simulink model "Scenario_13_CoDeSys"  (R2012b)
settings: Solver=ode3  StartTime=0.0  StopTime=inf  FixedStep=Sample_Time_Model  RelTol=1e-3
PreLoadFcn:
  | Variablen_Scenario13
InitFcn:
  | BT = randperm(9);
values from neighbouring files (symbols this model uses):
  Band_Geschwindigkeit = 1.47    [Variablen_Scenario13.m]
  Band_Sensor_Hell_2_Z = -6.5    [Variablen_Scenario13.m]
  Band_Sensor_Hell_3_Z = -10.36    [Variablen_Scenario13.m]
  Band_Sensor_Hell_4_Z = -14.64    [Variablen_Scenario13.m]
  Band_Sensor_Tolerance_Z = 0.2    [Variablen_Scenario13.m]
  Bauteil_Fallgeschwindigkeit = 0.4    [Variablen_Scenario13.m]
  Bauteil_Farbe_Metall = [0.8 0.8 0.8]    [Variablen_Scenario13.m]
  Bauteil_Farbe_Schwarz = [0.2 0.2 0.2]    [Variablen_Scenario13.m]
  Bauteil_Farbe_Weiss = [1 1 0.2]    [Variablen_Scenario13.m]
  Kran_Dauer_90_Grad = 5    [Variablen_Scenario13.m]
  Kran_Drehwinkel_90_Grad = 8050    [Variablen_Scenario13.m]
  Kran_Sensor_Position_Delta = 0.07    [Variablen_Scenario13.m]
  Sample_Time_Model = 0.05    [Variablen_Scenario13.m]
  Sample_Time_Simulation = 0.1    [Variablen_Scenario13.m]
  Sensor_Band_Metall_1 = -6.5    [Variablen_Scenario13.m]
  Sensor_Band_Metall_2 = -10.36    [Variablen_Scenario13.m]
libraries: simulink x557, vrlib x13, opclib x7, rtwinlib x1
(part 5 of 10)

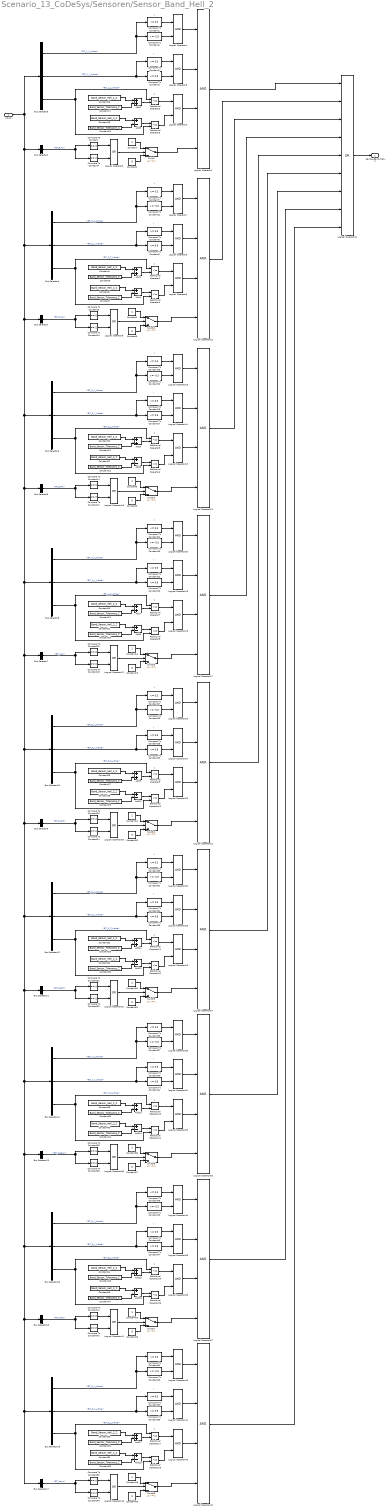
== system Scenario_13_CoDeSys/Sensoren/Sensor_Band_Hell_2 ==
  note: Y
  note: X
  note: Z
  note: Y
  note: X
  note: Z
  note: Y
  note: X
  note: Z
  note: Y
  note: X
  note: Z
  note: Y
  note: X
  note: Z
  note: Y
  note: X
  note: Z
  note: Y
  note: Z
  note: Y
  note: Z
  note: Y
  note: Z
  Inputs : Inport
  Add{1..2,5,7,9,11,13,15,17} (9 alike) : Sum
  Add{3..4,6,8,10,12,14,16,18} (9 alike) : Sum  Inputs=+-
  Bus Selector1 : BusSelector  OutputSignals=Eingaenge.Bauteile.BT_Zwei
  Bus Selector10 : BusSelector  OutputSignals=Bauteil.Stempelanlage_BT.Bauteil_5.BT_5_X_Achse,Bauteil.Stempelanlage_BT.Bauteil_5.BT_5_Y_Achse,Bauteil.Stempelanlage_BT.Bauteil_5.BT_5_Z_Achse
  Bus Selector11 : BusSelector  OutputSignals=Eingaenge.Bauteile.BT_Sechs
  Bus Selector12 : BusSelector  OutputSignals=Bauteil.Stempelanlage_BT.Bauteil_6.BT_6_X_Achse,Bauteil.Stempelanlage_BT.Bauteil_6.BT_6_Y_Achse,Bauteil.Stempelanlage_BT.Bauteil_6.BT_6_Z_Achse
  Bus Selector13 : BusSelector  OutputSignals=Eingaenge.Bauteile.BT_Sieben
  Bus Selector14 : BusSelector  OutputSignals=Bauteil.Stempelanlage_BT.Bauteil_7.BT_7_X_Achse,Bauteil.Stempelanlage_BT.Bauteil_7.BT_7_Y_Achse,Bauteil.Stempelanlage_BT.Bauteil_7.BT_7_Z_Achse
  Bus Selector15 : BusSelector  OutputSignals=Eingaenge.Bauteile.BT_Acht
  Bus Selector16 : BusSelector  OutputSignals=Bauteil.Stempelanlage_BT.Bauteil_8.BT_8_X_Achse,Bauteil.Stempelanlage_BT.Bauteil_8.BT_8_Y_Achse,Bauteil.Stempelanlage_BT.Bauteil_8.BT_8_Z_Achse
  Bus Selector17 : BusSelector  OutputSignals=Eingaenge.Bauteile.BT_Neun
  Bus Selector18 : BusSelector  OutputSignals=Bauteil.Stempelanlage_BT.Bauteil_9.BT_9_X_Achse,Bauteil.Stempelanlage_BT.Bauteil_9.BT_9_Y_Achse,Bauteil.Stempelanlage_BT.Bauteil_9.BT_9_Z_Achse
  Bus Selector2 : BusSelector  OutputSignals=Eingaenge.Bauteile.BT_Eins
  Bus Selector3 : BusSelector  OutputSignals=Bauteil.Stempelanlage_BT.Bauteil_1.BT_1_X_Achse,Bauteil.Stempelanlage_BT.Bauteil_1.BT_1_Y_Achse,Bauteil.Stempelanlage_BT.Bauteil_1.BT_1_Z_Achse
  Bus Selector4 : BusSelector  OutputSignals=Bauteil.Stempelanlage_BT.Bauteil_2.BT_2_X_Achse,Bauteil.Stempelanlage_BT.Bauteil_2.BT_2_Y_Achse,Bauteil.Stempelanlage_BT.Bauteil_2.BT_2_Z_Achse
  Bus Selector5 : BusSelector  OutputSignals=Eingaenge.Bauteile.BT_Drei
  Bus Selector6 : BusSelector  OutputSignals=Bauteil.Stempelanlage_BT.Bauteil_3.BT_3_X_Achse,Bauteil.Stempelanlage_BT.Bauteil_3.BT_3_Y_Achse,Bauteil.Stempelanlage_BT.Bauteil_3.BT_3_Z_Achse
  Bus Selector7 : BusSelector  OutputSignals=Eingaenge.Bauteile.BT_Vier
  Bus Selector8 : BusSelector  OutputSignals=Bauteil.Stempelanlage_BT.Bauteil_4.BT_4_X_Achse,Bauteil.Stempelanlage_BT.Bauteil_4.BT_4_Y_Achse,Bauteil.Stempelanlage_BT.Bauteil_4.BT_4_Z_Achse
  Bus Selector9 : BusSelector  OutputSignals=Eingaenge.Bauteile.BT_Fuenf
  Compare To Constant{,5,14,20,26,32,38,44,50} (9 alike) : simulink/Logic and Bit Operations/Compare To Constant  relop===  const=0  OutDataTypeStr=boolean
  Compare To Constant{1,7,15,21,27,33,39,45,51} (9 alike) : simulink/Logic and Bit Operations/Compare To Constant  relop=<=  const=0.3  OutDataTypeStr=boolean
  Compare To Constant{4,10,12,18,24,30,36,42,48} (9 alike) : simulink/Logic and Bit Operations/Compare To Constant  relop===  const=2  OutDataTypeStr=boolean
  Compare To Constant{6,11,13,19,25,31,37,43,49} (9 alike) : simulink/Logic and Bit Operations/Compare To Constant  relop=>=  const=-0.3  OutDataTypeStr=boolean
  Compare To Constant{2,8,16,22,28,34,40,46,52} (9 alike) : simulink/Logic and Bit Operations/Compare To Constant  relop=>=  const=0.5  OutDataTypeStr=boolean
  Compare To Constant{3,9,17,23,29,35,41,47,53} (9 alike) : simulink/Logic and Bit Operations/Compare To Constant  relop=<=  const=0.9  OutDataTypeStr=boolean
  Constant{,2,8,14,24,30,36,42,48} (9 alike) : Constant
  Constant{1,3,9,15,25,31,37,43,49} (9 alike) : Constant  Value=0
  Constant{4,6,10,12,16,18,20,22,26,28,32,34,38,40,44,46,50,52} (18 alike) : Constant  Value=Band_Sensor_Hell_2_Z
  Constant{5,7,11,13,17,19,21,23,27,29,33,35,39,41,45,47,51,53} (18 alike) : Constant  Value=Band_Sensor_Tolerance_Z
  Logical Operator{1,10,12,17,22,27,32,37,42} (9 alike) : Logic  Inputs=4  AllPortsSameDT=off  OutDataTypeStr=boolean
  Logical Operator11 : Logic  Operator=OR  Inputs=9  AllPortsSameDT=off  OutDataTypeStr=boolean
  Logical Operator{2..7,13..15,18..20,23..25,28..30,33..35,38..40,43..45} (27 alike) : Logic  AllPortsSameDT=off  OutDataTypeStr=boolean
  Logical Operator{8..9,16,21,26,31,36,41,46} (9 alike) : Logic  Operator=OR  AllPortsSameDT=off  OutDataTypeStr=boolean
  Relational Operator{1..18} (18 alike) : RelationalOperator  Operator=<=  OutDataTypeStr=boolean
  Switch{,1..8} (9 alike) : Switch  Threshold=1
  Sensor_Band_Hell_2 : Outport
  wires:
  Bus Selector3/2 -> Compare To Constant2/1, Compare To Constant3/1  "<BT_1_Y_Achse>"
  Compare To Constant2/1 -> Logical Operator3/1
  Compare To Constant3/1 -> Logical Operator3/2
  Logical Operator3/1 -> Logical Operator1/2
  Logical Operator2/1 -> Logical Operator1/3
  Bus Selector3/1 -> Compare To Constant1/1, Compare To Constant6/1  "<BT_1_X_Achse>"
  Compare To Constant1/1 -> Logical Operator4/1
  Compare To Constant6/1 -> Logical Operator4/2
  Logical Operator4/1 -> Logical Operator1/1
  Bus Selector2/1 -> Compare To Constant/1, Compare To Constant4/1  "<BT_Eins>"
  Constant/1 -> Switch/1
  Constant1/1 -> Switch/3
  Relational Operator2/1 -> Logical Operator2/1
  Constant16/1 -> Add2/1
  Constant17/1 -> Add2/2
  Constant18/1 -> Add3/1
  Constant19/1 -> Add3/2
  Add2/1 -> Relational Operator2/2
  Add3/1 -> Relational Operator3/1
  Bus Selector3/3 -> Relational Operator2/1, Relational Operator3/2  "<BT_1_Z_Achse>"
  Relational Operator3/1 -> Logical Operator2/2
  Compare To Constant/1 -> Logical Operator9/1
  Compare To Constant4/1 -> Logical Operator9/2
  Logical Operator9/1 -> Switch/2
  Switch/1 -> Logical Operator1/4
  Compare To Constant8/1 -> Logical Operator6/1
  Compare To Constant9/1 -> Logical Operator6/2
  Logical Operator6/1 -> Logical Operator10/2
  Logical Operator5/1 -> Logical Operator10/3
  Bus Selector4/1 -> Compare To Constant7/1, Compare To Constant11/1  "<BT_2_X_Achse>"
  Compare To Constant7/1 -> Logical Operator7/1
  Compare To Constant11/1 -> Logical Operator7/2
  Logical Operator7/1 -> Logical Operator10/1
  Bus Selector1/1 -> Compare To Constant5/1, Compare To Constant10/1  "<BT_Zwei>"
  Constant2/1 -> Switch1/1
  Constant3/1 -> Switch1/3
  Relational Operator1/1 -> Logical Operator5/1
  Constant4/1 -> Add1/1
  Constant5/1 -> Add1/2
  Constant6/1 -> Add4/1
  Constant7/1 -> Add4/2
  Add1/1 -> Relational Operator1/2
  Add4/1 -> Relational Operator4/1
  Bus Selector4/3 -> Relational Operator1/1, Relational Operator4/2  "<BT_2_Z_Achse>"
  Relational Operator4/1 -> Logical Operator5/2
  Compare To Constant5/1 -> Logical Operator8/1
  Compare To Constant10/1 -> Logical Operator8/2
  Logical Operator8/1 -> Switch1/2
  Switch1/1 -> Logical Operator10/4
  Bus Selector4/2 -> Compare To Constant8/1, Compare To Constant9/1  "<BT_2_Y_Achse>"
  Logical Operator11/1 -> Sensor_Band_Hell_2/1
  Logical Operator1/1 -> Logical Operator11/1
  Logical Operator10/1 -> Logical Operator11/2
  Compare To Constant16/1 -> Logical Operator14/1
  Compare To Constant17/1 -> Logical Operator14/2
  Logical Operator14/1 -> Logical Operator12/2
  Logical Operator13/1 -> Logical Operator12/3
  Bus Selector6/1 -> Compare To Constant15/1, Compare To Constant13/1  "<BT_3_X_Achse>"
  Compare To Constant15/1 -> Logical Operator15/1
  Compare To Constant13/1 -> Logical Operator15/2
  Logical Operator15/1 -> Logical Operator12/1
  Bus Selector5/1 -> Compare To Constant14/1, Compare To Constant12/1  "<BT_Drei>"
  Constant8/1 -> Switch2/1
  Constant9/1 -> Switch2/3
  Relational Operator5/1 -> Logical Operator13/1
  Constant10/1 -> Add5/1
  Constant11/1 -> Add5/2
  Constant12/1 -> Add6/1
  Constant13/1 -> Add6/2
  Add5/1 -> Relational Operator5/2
  Add6/1 -> Relational Operator6/1
  Bus Selector6/3 -> Relational Operator5/1, Relational Operator6/2  "<BT_3_Z_Achse>"
  Relational Operator6/1 -> Logical Operator13/2
  Compare To Constant14/1 -> Logical Operator16/1
  Compare To Constant12/1 -> Logical Operator16/2
  Logical Operator16/1 -> Switch2/2
  Switch2/1 -> Logical Operator12/4
  Bus Selector6/2 -> Compare To Constant16/1, Compare To Constant17/1  "<BT_3_Y_Achse>"
  Compare To Constant22/1 -> Logical Operator19/1
  Compare To Constant23/1 -> Logical Operator19/2
  Logical Operator19/1 -> Logical Operator17/2
  Logical Operator18/1 -> Logical Operator17/3
  Bus Selector8/1 -> Compare To Constant21/1, Compare To Constant19/1  "<BT_4_X_Achse>"
  Compare To Constant21/1 -> Logical Operator20/1
  Compare To Constant19/1 -> Logical Operator20/2
  Logical Operator20/1 -> Logical Operator17/1
  Bus Selector7/1 -> Compare To Constant20/1, Compare To Constant18/1  "<BT_Vier>"
  Constant14/1 -> Switch3/1
  Constant15/1 -> Switch3/3
  Relational Operator7/1 -> Logical Operator18/1
  Constant20/1 -> Add7/1
  Constant21/1 -> Add7/2
  Constant22/1 -> Add8/1
  Constant23/1 -> Add8/2
  Add7/1 -> Relational Operator7/2
  Add8/1 -> Relational Operator8/1
  Bus Selector8/3 -> Relational Operator7/1, Relational Operator8/2  "<BT_4_Z_Achse>"
  Relational Operator8/1 -> Logical Operator18/2
  Compare To Constant20/1 -> Logical Operator21/1
  Compare To Constant18/1 -> Logical Operator21/2
  Logical Operator21/1 -> Switch3/2
  Switch3/1 -> Logical Operator17/4
  Bus Selector8/2 -> Compare To Constant22/1, Compare To Constant23/1  "<BT_4_Y_Achse>"
  Compare To Constant28/1 -> Logical Operator24/1
  Compare To Constant29/1 -> Logical Operator24/2
  Logical Operator24/1 -> Logical Operator22/2
  Logical Operator23/1 -> Logical Operator22/3
  Bus Selector10/1 -> Compare To Constant27/1, Compare To Constant25/1  "<BT_5_X_Achse>"
  Compare To Constant27/1 -> Logical Operator25/1
  Compare To Constant25/1 -> Logical Operator25/2
  Logical Operator25/1 -> Logical Operator22/1
  Bus Selector9/1 -> Compare To Constant26/1, Compare To Constant24/1  "<BT_Fuenf>"
  Constant24/1 -> Switch4/1
  Constant25/1 -> Switch4/3
  Relational Operator9/1 -> Logical Operator23/1
  Constant26/1 -> Add9/1
  Constant27/1 -> Add9/2
  Constant28/1 -> Add10/1
  Constant29/1 -> Add10/2
  Add9/1 -> Relational Operator9/2
  Add10/1 -> Relational Operator10/1
  Bus Selector10/3 -> Relational Operator9/1, Relational Operator10/2  "<BT_5_Z_Achse>"
  Relational Operator10/1 -> Logical Operator23/2
  Compare To Constant26/1 -> Logical Operator26/1
  Compare To Constant24/1 -> Logical Operator26/2
  Logical Operator26/1 -> Switch4/2
  Switch4/1 -> Logical Operator22/4
  Bus Selector10/2 -> Compare To Constant28/1, Compare To Constant29/1  "<BT_5_Y_Achse>"
  Compare To Constant34/1 -> Logical Operator29/1
  Compare To Constant35/1 -> Logical Operator29/2
  Logical Operator29/1 -> Logical Operator27/2
  Logical Operator28/1 -> Logical Operator27/3
  Bus Selector12/1 -> Compare To Constant33/1, Compare To Constant31/1  "<BT_6_X_Achse>"
  Compare To Constant33/1 -> Logical Operator30/1
  Compare To Constant31/1 -> Logical Operator30/2
  Logical Operator30/1 -> Logical Operator27/1
  Bus Selector11/1 -> Compare To Constant32/1, Compare To Constant30/1  "<BT_Sechs>"
  Constant30/1 -> Switch5/1
  Constant31/1 -> Switch5/3
  Relational Operator11/1 -> Logical Operator28/1
  Constant32/1 -> Add11/1
  Constant33/1 -> Add11/2
  Constant34/1 -> Add12/1
  Constant35/1 -> Add12/2
  Add11/1 -> Relational Operator11/2
  Add12/1 -> Relational Operator12/1
  Bus Selector12/3 -> Relational Operator11/1, Relational Operator12/2  "<BT_6_Z_Achse>"
  Relational Operator12/1 -> Logical Operator28/2
  Compare To Constant32/1 -> Logical Operator31/1
  Compare To Constant30/1 -> Logical Operator31/2
  Logical Operator31/1 -> Switch5/2
  Switch5/1 -> Logical Operator27/4
  Bus Selector12/2 -> Compare To Constant34/1, Compare To Constant35/1  "<BT_6_Y_Achse>"
  Logical Operator12/1 -> Logical Operator11/3
  Logical Operator17/1 -> Logical Operator11/4
  Logical Operator22/1 -> Logical Operator11/5
  Logical Operator27/1 -> Logical Operator11/6
  Inputs/1 -> Bus Selector6/1, Bus Selector5/1, Bus Selector8/1, Bus Selector7/1, Bus Selector10/1, Bus Selector9/1, Bus Selector12/1, Bus Selector14/1, Bus Selector13/1, Bus Selector16/1, Bus Selector15/1, Bus Selector18/1, Bus Selector17/1, Bus Selector11/1, Bus Selector1/1, Bus Selector4/1, Bus Selector2/1, Bus Selector3/1
  Compare To Constant40/1 -> Logical Operator34/1
  Compare To Constant41/1 -> Logical Operator34/2
  Logical Operator34/1 -> Logical Operator32/2
  Logical Operator33/1 -> Logical Operator32/3
  Bus Selector14/1 -> Compare To Constant39/1, Compare To Constant37/1  "<BT_7_X_Achse>"
  Compare To Constant39/1 -> Logical Operator35/1
  Compare To Constant37/1 -> Logical Operator35/2
  Logical Operator35/1 -> Logical Operator32/1
  Bus Selector13/1 -> Compare To Constant38/1, Compare To Constant36/1  "<BT_Sieben>"
  Constant36/1 -> Switch6/1
  Constant37/1 -> Switch6/3
  Relational Operator13/1 -> Logical Operator33/1
  Constant38/1 -> Add13/1
  Constant39/1 -> Add13/2
  Constant40/1 -> Add14/1
  Constant41/1 -> Add14/2
  Add13/1 -> Relational Operator13/2
  Add14/1 -> Relational Operator14/1
  Bus Selector14/3 -> Relational Operator13/1, Relational Operator14/2  "<BT_7_Z_Achse>"
  Relational Operator14/1 -> Logical Operator33/2
  Compare To Constant38/1 -> Logical Operator36/1
  Compare To Constant36/1 -> Logical Operator36/2
  Logical Operator36/1 -> Switch6/2
  Switch6/1 -> Logical Operator32/4
  Bus Selector14/2 -> Compare To Constant40/1, Compare To Constant41/1  "<BT_7_Y_Achse>"
  Compare To Constant46/1 -> Logical Operator39/1
  Compare To Constant47/1 -> Logical Operator39/2
  Logical Operator39/1 -> Logical Operator37/2
  Logical Operator38/1 -> Logical Operator37/3
  Bus Selector16/1 -> Compare To Constant45/1, Compare To Constant43/1  "<BT_8_X_Achse>"
  Compare To Constant45/1 -> Logical Operator40/1
  Compare To Constant43/1 -> Logical Operator40/2
  Logical Operator40/1 -> Logical Operator37/1
  Bus Selector15/1 -> Compare To Constant44/1, Compare To Constant42/1  "<BT_Acht>"
  Constant42/1 -> Switch7/1
  Constant43/1 -> Switch7/3
  Relational Operator15/1 -> Logical Operator38/1
  Constant44/1 -> Add15/1
  Constant45/1 -> Add15/2
  Constant46/1 -> Add16/1
  Constant47/1 -> Add16/2
  Add15/1 -> Relational Operator15/2
  Add16/1 -> Relational Operator16/1
  Bus Selector16/3 -> Relational Operator15/1, Relational Operator16/2  "<BT_8_Z_Achse>"
  Relational Operator16/1 -> Logical Operator38/2
  Compare To Constant44/1 -> Logical Operator41/1
  Compare To Constant42/1 -> Logical Operator41/2
  Logical Operator41/1 -> Switch7/2
  Switch7/1 -> Logical Operator37/4
  Bus Selector16/2 -> Compare To Constant46/1, Compare To Constant47/1  "<BT_8_Y_Achse>"
  Compare To Constant52/1 -> Logical Operator44/1
  Compare To Constant53/1 -> Logical Operator44/2
  Logical Operator44/1 -> Logical Operator42/2
  Logical Operator43/1 -> Logical Operator42/3
  Bus Selector18/1 -> Compare To Constant51/1, Compare To Constant49/1  "<BT_9_X_Achse>"
  Compare To Constant51/1 -> Logical Operator45/1
  Compare To Constant49/1 -> Logical Operator45/2
  Logical Operator45/1 -> Logical Operator42/1
  Bus Selector17/1 -> Compare To Constant48/1, Compare To Constant50/1  "<BT_Neun>"
  Constant48/1 -> Switch8/1
  Constant49/1 -> Switch8/3
  Relational Operator17/1 -> Logical Operator43/1
  Constant50/1 -> Add17/1
  Constant51/1 -> Add17/2
  Constant52/1 -> Add18/1
  Constant53/1 -> Add18/2
  Add17/1 -> Relational Operator17/2
  Add18/1 -> Relational Operator18/1
  Bus Selector18/3 -> Relational Operator17/1, Relational Operator18/2  "<BT_9_Z_Achse>"
  Relational Operator18/1 -> Logical Operator43/2
  Compare To Constant50/1 -> Logical Operator46/1
  Compare To Constant48/1 -> Logical Operator46/2
  Logical Operator46/1 -> Switch8/2
  Switch8/1 -> Logical Operator42/4
  Bus Selector18/2 -> Compare To Constant52/1, Compare To Constant53/1  "<BT_9_Y_Achse>"
  Logical Operator32/1 -> Logical Operator11/7
  Logical Operator37/1 -> Logical Operator11/8
  Logical Operator42/1 -> Logical Operator11/9

== stateflow chart Scenario_13_CoDeSys/Signal Expander/Band_Zyl_1 ==
  state Schrittgroesse [function]
    (default) -> (junction 106) : {Schrittgroesse = (3* Sample_Time)/0.11}
  state Berechne_Naechste_Position_Einfahren [function]
    (default) -> (junction 134) : {Naechste_Position = Zyl_1_X_Achse - Schrittgroesse;}
    (junction 134) -> (junction 135) [order 1] : [Naechste_Position <= -1]
    (junction 134) -> (junction 136) [order 2] : {Zyl_1_X_Achse = Naechste_Position;}
    (junction 135) -> (junction 137) : {Zyl_1_X_Achse = -1;}
    (junction 137) -> (junction 136)
  state Zyl_1_Bereit
    entry: Zyl_1_X_Achse = -1;
    Band_Zyl_1_Eingefahren = 1;
    exit: Band_Zyl_1_Eingefahren = 0;
  state Berechne_Naechste_Position_Ausfahren [function]
    (default) -> (junction 124) : {Naechste_Position = Zyl_1_X_Achse + Schrittgroesse;}
    (junction 124) -> (junction 125) [order 1] : [Naechste_Position >= 2]
    (junction 124) -> (junction 126) [order 2] : {Zyl_1_X_Achse = Naechste_Position;}
    (junction 125) -> (junction 127) : {Zyl_1_X_Achse = 2;}
    (junction 127) -> (junction 126)
  state r = Stop_Einfahren [function]
    (default) -> (junction 198) : {r=0}
    (junction 198) -> (junction 199) [order 1] : [!Zyl_1_Einfahren || (Zyl_1_Ausfahren && Zyl_1_Einfahren)]
    (junction 199) -> (junction 201) : {r=1}
    (junction 198) -> (junction 200) [order 2]
    (junction 201) -> (junction 200)
  state Stop
  state Zyl_1_Ausfahren
    during: Berechne_Naechste_Position_Ausfahren();
  state r = Stop_Ausfahren [function]
    (default) -> (junction 209) : {r=0}
    (junction 209) -> (junction 210) [order 1] : [!Zyl_1_Ausfahren || (Zyl_1_Ausfahren && Zyl_1_Einfahren)]
    (junction 210) -> (junction 212) : {r=1}
    (junction 209) -> (junction 211) [order 2]
    (junction 212) -> (junction 211)
  state r = Continue_Einfahren [function]
    (default) -> (junction 187) : {r=0}
    (junction 187) -> (junction 188) [order 1] : [Zyl_1_Einfahren && !Zyl_1_Ausfahren]
    (junction 188) -> (junction 190) : {r=1}
    (junction 187) -> (junction 189) [order 2]
    (junction 190) -> (junction 189)
  state Zyl_1_Ausgefahren
    entry: Band_Zyl_1_Ausgefahren = 1;
    Zyl_1_X_Achse = 2;
    exit: Band_Zyl_1_Ausgefahren = 0;
  state r = Continue_Ausfahren [function]
    (default) -> (junction 176) : {r=0}
    (junction 176) -> (junction 177) [order 1] : [Zyl_1_Ausfahren && !Zyl_1_Einfahren]
    (junction 177) -> (junction 179) : {r=1}
    (junction 176) -> (junction 178) [order 2]
    (junction 179) -> (junction 178)
  state Zyl_1_Einfahren
    during: Berechne_Naechste_Position_Einfahren();
  (default) -> Zyl_1_Bereit : {Schrittgroesse();}
  Zyl_1_Bereit -> Zyl_1_Ausfahren : [Zyl_1_Ausfahren && !Zyl_1_Einfahren]
  Zyl_1_Einfahren -> Zyl_1_Bereit [order 1] : [Zyl_1_X_Achse <= -1]
  Zyl_1_Ausfahren -> Stop [order 2] : [Stop_Ausfahren()]
  Stop -> Zyl_1_Ausfahren [order 1] : [Continue_Ausfahren()]
  Stop -> Zyl_1_Einfahren [order 2] : [Continue_Einfahren()]
  Zyl_1_Einfahren -> Stop [order 2] : [Stop_Einfahren()]
  Zyl_1_Ausfahren -> Zyl_1_Ausgefahren [order 1] : [Zyl_1_X_Achse >= 2]
  Zyl_1_Ausgefahren -> Zyl_1_Einfahren : [Zyl_1_Einfahren && !Zyl_1_Ausfahren]
  data: r function_output double; r function_output double; r function_output double; r function_output double; Zyl_1_Einfahren input; Zyl_1_X_Achse output double; Zyl_1_Ausfahren input; Band_Zyl_1_Eingefahren output double; Band_Zyl_1_Ausgefahren output double; Sample_Time input; Schrittgroesse output double; Naechste_Position local double

== stateflow chart Scenario_13_CoDeSys/Signal Expander/Kran_Sauger ==
  state Kran_Sauger_AN
    entry: Kran_Sauger_On = 1;
  state Kran_Sauger_Aus
    entry: Kran_Sauger_On = 0;
  Kran_Sauger_Aus -> Kran_Sauger_AN : [Kran_Sauger_An && !Kran_Sauger_Aus]
  (default) -> Kran_Sauger_Aus
  Kran_Sauger_AN -> Kran_Sauger_Aus : [Kran_Sauger_Aus || !Kran_Sauger_An]
  data: Kran_Sauger_An input; Kran_Sauger_Aus input; Kran_Sauger_On output double

== stateflow chart Scenario_13_CoDeSys/Signal Expander/Bauteil_9 ==
  state Bauteil_Pos_9
    entry:
    BT_X_Achse = 5.75;
    BT_Y_Achse = 8.9;
    x =0;
  state Bauteil_Faellt5
    during:
    BT_Y_Achse = Next_Pos_Minus_Min(BT_Y_Achse, Bauteil_Fallgeschwindigkeit, 7.87);
  state Bauteil_Pos_8
    entry:
    BT_X_Achse = 5.75;
    BT_Y_Achse = 7.87;
    x =0;
  state Bauteil_Faellt4
    during:
    BT_Y_Achse = Next_Pos_Minus_Min(BT_Y_Achse, Bauteil_Fallgeschwindigkeit, 6.84);
  state Bauteil_Pos_7
    entry:
    BT_X_Achse = 5.75;
    BT_Y_Achse = 6.84;
    x =0;
  state Bauteil_Faellt3
    during:
    BT_Y_Achse = Next_Pos_Minus_Min(BT_Y_Achse, Bauteil_Fallgeschwindigkeit, 5.83);
  state Bauteil_Pos_6
    entry:
    BT_X_Achse = 5.75;
    BT_Y_Achse = 5.81;
    x =0;
  state Bauteil_Faellt2
    during:
    BT_Y_Achse = Next_Pos_Minus_Min(BT_Y_Achse, Bauteil_Fallgeschwindigkeit, 4.8);
  state Stop1
  state Bauteil_Pos_2
  state Bauteil_Unten
  state Bauteil_Pos_5
  state Bauteil_Faellt_3
    during:
    BT_Y_Achse = Next_Pos_Minus_Min(BT_Y_Achse, Bauteil_Fallgeschwindigkeit, 0.7);
  state Drehen_Rechts_Runter [function]
    (default) -> (junction 322) : {BT_Y_Achse = Next_Pos_Minus_Min(BT_Y_Achse, Kran_Zyl_Schritt_Runter, 0.65);
        | x = x - Kran_Drehen_Schritt;
        | BT_Z_Achse = -3.5*sin(x);
        | BT_X_Achse = 3.5*cos(x);}
  state Bauteil_Faellt1
    during:
    BT_Y_Achse = Next_Pos_Minus_Min(BT_Y_Achse, Bauteil_Fallgeschwindigkeit, 3.77);
  state Drehen_Rechts_Hoch [function]
    (default) -> (junction 325) : {BT_Y_Achse = Next_Pos_Plus_Max(BT_Y_Achse, Kran_Zyl_Schritt_Hoch, 1.65);
        | x = x - Kran_Drehen_Schritt;
        | BT_Z_Achse = -3.5*sin(x);
        | BT_X_Achse = 3.5*cos(x);}
  state Bauteil_Lager_Vereinz_Ausfahren
    during:
    BT_X_Achse = BT_X_Achse - Lager_Vereinzler_Schritt_Aus;
  state Bauteil_Lager_Bereit
    entry: BT_Bereit = 1;
    BT_X_Achse = 3.5;
  state Drehen_Links_Runter [function]
    (default) -> (junction 319) : {BT_Y_Achse = Next_Pos_Minus_Min(BT_Y_Achse, Kran_Zyl_Schritt_Runter, 0.65);
        | x = x + Kran_Drehen_Schritt;
        | BT_Z_Achse = -3.5*sin(x);
        | BT_X_Achse = 3.5*cos(x);}
  state Drehen_Links_Hoch [function]
    (default) -> (junction 309) : {BT_Y_Achse = Next_Pos_Plus_Max(BT_Y_Achse, Kran_Zyl_Schritt_Hoch, 1.65);
        | x = x + Kran_Drehen_Schritt;
        | BT_Z_Achse = -3.5*sin(x);
        | BT_X_Achse = 3.5*cos(x);}
  state Ausgabe = Next_Pos_Plus_Max(Achse, Schrittgroesse, MaxWert) [function]
    (default) -> (junction 249) : {Naechste_Position = Achse + Schrittgroesse;}
    (junction 249) -> (junction 250) [order 1] : [Naechste_Position >= MaxWert]
    (junction 249) -> (junction 251) [order 2] : {Ausgabe = Naechste_Position;}
    (junction 250) -> (junction 252) : {Ausgabe = MaxWert;}
    (junction 252) -> (junction 251)
  state Bauteil_Pos_3
  state Bauteil_Kran_Hochheben_Bereit
    entry: BT_Bereit = 1;
    Kran_Sauger_BT = 1;
  state Bauteil_Faellt_2
    during:
    BT_Y_Achse = Next_Pos_Minus_Min(BT_Y_Achse, Bauteil_Fallgeschwindigkeit, 1.73);
  state Bauteil_Pos_4
  state Bauteil_Faellt
    during:
    BT_Y_Achse = Next_Pos_Minus_Min(BT_Y_Achse, Bauteil_Fallgeschwindigkeit, 2.75);
  state Ausgabe = Next_Pos_Minus_Min(Achse, Schrittgroesse, MinWert) [function]
    (default) -> (junction 268) : {Naechste_Position = Achse - Schrittgroesse;}
    (junction 268) -> (junction 269) [order 1] : [Naechste_Position <= MinWert]
    (junction 268) -> (junction 270) [order 2] : {Ausgabe = Naechste_Position;}
    (junction 269) -> (junction 271) : {Ausgabe = MinWert;}
    (junction 271) -> (junction 270)
  state Ausgabe = Lager_Y_Achse(Lager_Status, Pos_1, Pos_2, Pos_3) [function]
    (default) -> (junction 412)
    (junction 412) -> (junction 411) [order 3] : [Lager_Status == 2]
    (junction 412) -> (junction 413) [order 1] : [Lager_Status == 0]
    (junction 411) -> (junction 414) : {Ausgabe = Pos_3;}
    (junction 412) -> (junction 415) [order 2] : [Lager_Status == 1]
        | {Ausgabe = Pos_2;}
    (junction 413) -> (junction 416) : {Ausgabe = Pos_1;}
    (junction 414) -> (junction 415)
    (junction 416) -> (junction 415)
  state Bauteil_Stempel_Halterung_Einfahren
    during:
    BT_X_Achse = Next_Pos_Minus_Min(BT_X_Achse, Stempel_Halterung_Schritt_Ein, -4.6);
  state Bauteil_Kran_Runterlassen
    during:
    BT_Y_Achse = Next_Pos_Minus_Min(BT_Y_Achse, Kran_Zyl_Schritt_Runter, 0.65);
  state Bauteil_Kran_Hochheben
    during:
    BT_Y_Achse = Next_Pos_Plus_Max(BT_Y_Achse, Kran_Zyl_Schritt_Hoch, 1.65);
  state Bauteil_Faellt_Auf_Festen_Untergrund
  state Bauteil_Lost
  state Bauteil_Lager_1_Ende
    entry: BT_Y_Achse = Lager_Y_Achse(Lager_1_Status, -0.158, 0.037, 0.232);
    BT_Lager = 1;
  state Bauteil_Abgesetzt_Stempel
    entry: Kran_Sauger_BT = 0;
  state Bauteil_Kran_Zyl_Stop
  state Bauteil_Stempel_Halterung_Stop
  state Drop_Down
    entry: Kran_Sauger_BT = 0;
    during:
    BT_Y_Achse = BT_Y_Achse - 0.4;
  state Bauteil_Lager_1_Beginnt
    entry: BT_Rotation_1 = 0;
    BT_Rotation_2 = 0;
    BT_Rotation_3 = 1;
    BT_Rotation_4 = 0.2;
    during:
    BT_X_Achse = Next_Pos_Minus_Min(BT_X_Achse, Band_Zyl_1_Schritt, -6.5 + Lager_1_Status);
    BT_Y_Achse = BT_Y_Achse - (0.2 * Band_Zyl_1_Schritt);
  state Bauteil_Stempel_Halterung_Ausfahren
    during:
    BT_X_Achse = Next_Pos_Plus_Max(BT_X_Achse, Stempel_Halterung_Schritt_Aus, -3.4);
  note: Bei -2,8 beginnt in etwa die Schraege !!
  state Drehen_Links
    during:
    x = x + Kran_Drehen_Schritt;
    BT_Z_Achse = -3.5*sin(x);
    BT_X_Achse = 3.5*cos(x);
  state Bauteil_Band_Vor
    during:
    BT_Z_Achse = BT_Z_Achse - Band_Geschwindigkeit;
  state Bauteil_Lager_1_Schieben
    during:
    BT_X_Achse = Next_Pos_Minus_Min(BT_X_Achse, Band_Zyl_1_Schritt, -2.7);
  state Bauteil_Lager_2_Ende
    entry: BT_Y_Achse = Lager_Y_Achse(Lager_2_Status, -0.158, 0.037, 0.232);
    BT_Lager = 2;
  state Bauteil_Kran_Rot_Stop
  state Bauteil_Band_Stop
    entry: Kran_Sauger_BT = 0;
  state Drehen_Rechts
    during:
    x = x - Kran_Drehen_Schritt;
    BT_Z_Achse = -3.5*sin(x);
    BT_X_Achse = 3.5*cos(x);
  state Bauteil_Lager_2_Beginnt
    entry: BT_Rotation_1 = 0;
    BT_Rotation_2 = 0;
    BT_Rotation_3 = 1;
    BT_Rotation_4 = 0.2;
    during:
    BT_X_Achse = Next_Pos_Minus_Min(BT_X_Achse, Band_Zyl_2_Schritt, -6.5 + Lager_2_Status);
    BT_Y_Achse = BT_Y_Achse - (0.2 * Band_Zyl_2_Schritt);
  state Bauteil_Band_Zurueck
    during:
    BT_Z_Achse = BT_Z_Achse + Band_Geschwindigkeit;
  state Bauteil_Lager_2_Schieben
    during:
    BT_X_Achse = Next_Pos_Minus_Min(BT_X_Achse, Band_Zyl_2_Schritt, -2.7);
  state Bauteil_Kran_Runterlassen_Und_Drehen_Rechts
    entry:
    x = x - Kran_Drehen_Schritt;
    BT_Z_Achse = -3.5*sin(x);
    BT_X_Achse = 3.5*cos(x);
    during: Drehen_Rechts_Runter();
  state Bauteil_Lager_3_Beginnt
    entry: BT_Rotation_1 = -1;
    BT_Rotation_2 = 0;
    BT_Rotation_3 = 0;
    BT_Rotation_4 = 0.2;
    during:
    BT_Z_Achse = Next_Pos_Minus_Min(BT_Z_Achse, 1.5 * Band_Geschwindigkeit, -19.05 + Lager_3_Status);
    BT_Y_Achse = BT_Y_Achse - (1.5 * 0.2*Band_Geschwindigkeit);
  state Bauteil_Kran_Hochheben_Und_Drehen_Links
    entry:
    x = x + Kran_Drehen_Schritt;
    BT_Z_Achse = -3.5*sin(x);
    BT_X_Achse = 3.5*cos(x);
    during: Drehen_Links_Hoch();
  state Bauteil_Lager_3_Ende
    entry: BT_Y_Achse = Lager_Y_Achse(Lager_3_Status, -0.158, 0.037, 0.232);
    BT_Lager = 3;
  state Bauteil_Kran_Hochheben_Und_Drehen_Rechts
    entry:
    x = x - Kran_Drehen_Schritt;
    BT_Z_Achse = -3.5*sin(x);
    BT_X_Achse = 3.5*cos(x);
    during:Drehen_Rechts_Hoch();
  state Bauteil_Kran_Runterlassen_Und_Drehen_Links
    entry:
    x = x + Kran_Drehen_Schritt;
    BT_Z_Achse = -3.5*sin(x);
    BT_X_Achse = 3.5*cos(x);
    during: Drehen_Links_Runter();
  (default) -> Bauteil_Pos_9
  Bauteil_Pos_9 -> Bauteil_Faellt5 : [BT_1_Bereit && Lager_Ver_Eingefahren]
  Bauteil_Faellt5 -> Bauteil_Pos_8 : [BT_Y_Achse <= 7.87]
  Bauteil_Pos_8 -> Bauteil_Faellt4 : [BT_2_Bereit && Lager_Ver_Eingefahren]
  Bauteil_Faellt4 -> Bauteil_Pos_7 : [BT_Y_Achse <= 6.84]
  Bauteil_Faellt_Auf_Festen_Untergrund -> Bauteil_Abgesetzt_Stempel [order 2] : [Kran_Stellung_Stempel]
  Bauteil_Pos_7 -> Bauteil_Faellt3 : [BT_3_Bereit && Lager_Ver_Eingefahren]
  Bauteil_Faellt3 -> Bauteil_Pos_6 : [BT_Y_Achse <= 5.83]
  Bauteil_Pos_6 -> Bauteil_Faellt2 : [BT_4_Bereit && Lager_Ver_Eingefahren]
  Bauteil_Faellt2 -> Bauteil_Pos_5 : [BT_Y_Achse <= 4.8]
  Stop1 -> Bauteil_Lager_Vereinz_Ausfahren : [BT_X_Achse + Lager_X_Achse >= 5.1]
  Bauteil_Lager_Vereinz_Ausfahren -> Stop1 [order 2] : [BT_X_Achse + Lager_X_Achse < 5.1]
  Bauteil_Pos_2 -> Bauteil_Faellt_3 : [BT_8_Bereit && Lager_Ver_Eingefahren]
  Bauteil_Unten -> Bauteil_Lager_Vereinz_Ausfahren : [Lager_Ver_Ausfahren && (BT_X_Achse + Lager_X_Achse >= 5.1)]
  Bauteil_Pos_5 -> Bauteil_Faellt1 : [BT_5_Bereit && Lager_Ver_Eingefahren]
  Bauteil_Faellt_2 -> Bauteil_Pos_2 : [BT_Y_Achse <= 1.73]
  Bauteil_Faellt_3 -> Bauteil_Unten : [BT_Y_Achse <= 0.7]
  Bauteil_Lager_Vereinz_Ausfahren -> Bauteil_Lager_Bereit [order 1] : [Lager_Ver_Ausgefahren]
  Bauteil_Faellt1 -> Bauteil_Pos_4 : [BT_Y_Achse <= 3.77]
  Bauteil_Faellt_Auf_Festen_Untergrund -> Bauteil_Lager_Bereit [order 1] : [Kran_Stellung_Lager]
  Bauteil_Lager_Bereit -> Bauteil_Kran_Hochheben_Bereit : [Kran_Stellung_Lager && Kran_Sauger && Kran_Zyl_Unten]
  Bauteil_Stempel_Halterung_Stop -> Bauteil_Kran_Hochheben_Bereit [order 3] : [Kran_Stellung_Stempel && Kran_Sauger && Kran_Zyl_Unten]
  (junction 127) -> Bauteil_Kran_Hochheben_Bereit [order 2] : [Kran_Stellung_Lager && Kran_Sauger && Kran_Zyl_Unten]
  Bauteil_Faellt -> Bauteil_Pos_3 : [BT_Y_Achse <= 2.75]
  Bauteil_Kran_Hochheben_Bereit -> Bauteil_Kran_Hochheben : [Kran_Hochheben]
      | {BT_Bereit = 0;}
  Bauteil_Pos_3 -> Bauteil_Faellt_2 : [BT_7_Bereit && Lager_Ver_Eingefahren]
  Bauteil_Pos_4 -> Bauteil_Faellt : [BT_6_Bereit && Lager_Ver_Eingefahren]
  Bauteil_Kran_Hochheben -> (junction 127) [order 3]
  Bauteil_Kran_Rot_Stop -> (junction 287) [order 4]
  (junction 287) -> Bauteil_Kran_Hochheben [order 2] : [Kran_Hochheben]
  (junction 287) -> Bauteil_Kran_Runterlassen [order 1] : [Kran_Runterlassen]
  Bauteil_Stempel_Halterung_Stop -> Bauteil_Stempel_Halterung_Einfahren [order 1] : [Stempel_Halterung_Einfahren]
  Bauteil_Stempel_Halterung_Einfahren -> Bauteil_Stempel_Halterung_Stop : [!Stempel_Halterung_Einfahren]
  Bauteil_Kran_Hochheben -> Bauteil_Kran_Runterlassen [order 1] : [Kran_Runterlassen]
  Bauteil_Kran_Runterlassen -> (junction 127) [order 2]
  Bauteil_Kran_Runterlassen -> (junction 162) [order 4]
  Bauteil_Kran_Zyl_Stop -> Bauteil_Kran_Runterlassen [order 3] : [Kran_Runterlassen]
  Bauteil_Kran_Runterlassen -> Bauteil_Kran_Zyl_Stop [order 3] : [Kran_Zyl_Unten]
  Bauteil_Kran_Runterlassen -> Bauteil_Kran_Hochheben [order 1] : [Kran_Hochheben]
  Drop_Down -> Bauteil_Lost [order 1] : [BT_Y_Achse <= -2]
  Bauteil_Kran_Hochheben -> (junction 162) [order 4]
  Bauteil_Kran_Hochheben -> Bauteil_Kran_Zyl_Stop [order 2] : [Kran_Zyl_Oben]
  Bauteil_Kran_Zyl_Stop -> Bauteil_Kran_Hochheben [order 2] : [Kran_Hochheben]
  Bauteil_Lager_1_Beginnt -> Bauteil_Lager_1_Ende : [BT_X_Achse <= (-6.5 + Lager_1_Status)]
  Drop_Down -> Bauteil_Faellt_Auf_Festen_Untergrund [order 2] : [(Kran_Stellung_Band || Kran_Stellung_Lager || Kran_Stellung_Stempel) && (BT_Y_Achse <= 0.65)]
  Bauteil_Abgesetzt_Stempel -> Bauteil_Stempel_Halterung_Stop
  Bauteil_Faellt_Auf_Festen_Untergrund -> Bauteil_Band_Stop [order 3] : [Kran_Stellung_Band]
  (junction 127) -> Drop_Down [order 1] : [!Kran_Sauger]
  Bauteil_Kran_Zyl_Stop -> (junction 127) [order 8]
  Drehen_Rechts -> Drop_Down [order 3] : [!Kran_Sauger]
  Bauteil_Kran_Zyl_Stop -> Bauteil_Abgesetzt_Stempel [order 6] : [Kran_Zyl_Unten && !Kran_Sauger && Kran_Stellung_Stempel]
  Bauteil_Stempel_Halterung_Ausfahren -> Bauteil_Stempel_Halterung_Stop : [!Stempel_Halterung_Ausfahren]
  Bauteil_Stempel_Halterung_Stop -> Bauteil_Stempel_Halterung_Ausfahren [order 2] : [Stempel_Halterung_Ausfahren]
  Bauteil_Kran_Rot_Stop -> Drop_Down [order 3] : [!Kran_Sauger]
  Drehen_Links -> Drop_Down [order 3] : [!Kran_Sauger]
  Bauteil_Kran_Zyl_Stop -> Drehen_Links [order 4] : [Kran_Drehen_Links]
  Bauteil_Kran_Zyl_Stop -> Drehen_Rechts [order 5] : [Kran_Drehen_Rechts]
  (junction 178) -> Bauteil_Kran_Zyl_Stop : [!Kran_Drehen_Rechts && !Kran_Drehen_Links]
  Bauteil_Kran_Zyl_Stop -> (junction 162) [order 1]
  Bauteil_Kran_Zyl_Stop -> Bauteil_Band_Stop [order 7] : [Kran_Zyl_Unten && !Kran_Sauger && Kran_Stellung_Band]
  Bauteil_Band_Stop -> Bauteil_Kran_Zyl_Stop [order 3] : [Kran_Zyl_Unten && Kran_Sauger && Kran_Stellung_Band && (-3.8 <= BT_Z_Achse) && (BT_Z_Achse <= -3.2) && (-0.3 <= BT_X_Achse) && (BT_X_Achse<= 0.3)]
  (junction 280) -> Drehen_Links [order 2] : [(Kran_Zyl_Unten || Kran_Zyl_Oben) && Kran_Drehen_Links]
      | {x = x + Kran_Drehen_Schritt;
      | BT_Z_Achse = -3.5*sin(x);
      | BT_X_Achse = 3.5*cos(x);}
  Drehen_Links -> Bauteil_Kran_Rot_Stop [order 2] : [!Kran_Drehen_Links]
  Bauteil_Lager_1_Schieben -> Bauteil_Lager_1_Beginnt : [BT_X_Achse <= -2.7]
  Bauteil_Kran_Rot_Stop -> Drehen_Links [order 1] : [Kran_Drehen_Links]
  Bauteil_Band_Vor -> (junction 135) [order 2]
  Drehen_Links -> (junction 162) [order 4]
  Drehen_Rechts -> Drehen_Links [order 1] : [Kran_Drehen_Links]
  Drehen_Links -> Drehen_Rechts [order 1] : [Kran_Drehen_Rechts]
  Bauteil_Band_Stop -> Bauteil_Band_Vor [order 1] : [Band_Vor]
  Bauteil_Band_Vor -> Bauteil_Band_Stop [order 1] : [!Band_Vor]
  (junction 135) -> Bauteil_Lager_1_Schieben [order 1] : [BT_Z_Achse <= -7.85 && BT_Z_Achse >= -8.65 && Band_Zyl_1_X_Achse >= -0.5]
  Bauteil_Lager_2_Beginnt -> Bauteil_Lager_2_Ende : [BT_X_Achse <= (-6.5 + Lager_2_Status)]
  (junction 280) -> Bauteil_Kran_Rot_Stop [order 3] : [Kran_Zyl_Unten || Kran_Zyl_Oben]
  Drehen_Rechts -> Bauteil_Kran_Rot_Stop [order 2] : [!Kran_Drehen_Rechts]
  Bauteil_Kran_Rot_Stop -> Drehen_Rechts [order 2] : [Kran_Drehen_Rechts]
  Bauteil_Band_Stop -> (junction 135) [order 4]
  (junction 135) -> Bauteil_Lager_2_Schieben [order 3] : [BT_Z_Achse <= -12.05 && BT_Z_Achse >= -12.85 && Band_Zyl_2_X_Achse >= -0.5]
  Bauteil_Band_Zurueck -> (junction 135) [order 2]
  (junction 135) -> Bauteil_Lager_3_Beginnt [order 2] : [BT_Z_Achse <= -14.6]
  Drehen_Rechts -> (junction 162) [order 4]
  Bauteil_Band_Zurueck -> Bauteil_Band_Stop [order 1] : [!Band_Zurueck]
  Bauteil_Band_Stop -> Bauteil_Band_Zurueck [order 2] : [Band_Zurueck]
  Bauteil_Kran_Runterlassen_Und_Drehen_Rechts -> (junction 178) [order 2]
  Bauteil_Kran_Hochheben_Und_Drehen_Links -> (junction 178) [order 2]
  Bauteil_Kran_Hochheben_Und_Drehen_Rechts -> (junction 178) [order 2]
  Bauteil_Kran_Runterlassen_Und_Drehen_Links -> (junction 178) [order 2]
  (junction 280) -> Drehen_Rechts [order 1] : [(Kran_Zyl_Unten || Kran_Zyl_Oben) && Kran_Drehen_Rechts]
      | {x = x - Kran_Drehen_Schritt;
      | BT_Z_Achse = -3.5*sin(x);
      | BT_X_Achse = 3.5*cos(x);}
  (junction 172) -> (junction 280)
  (junction 162) -> Bauteil_Kran_Runterlassen_Und_Drehen_Rechts [order 4] : [Kran_Drehen_Rechts && Kran_Runterlassen]
  (junction 162) -> Bauteil_Kran_Hochheben_Und_Drehen_Rechts [order 2] : [Kran_Drehen_Rechts && Kran_Hochheben]
  (junction 162) -> Bauteil_Kran_Hochheben_Und_Drehen_Links [order 1] : [Kran_Drehen_Links  && Kran_Hochheben]
  (junction 162) -> Bauteil_Kran_Runterlassen_Und_Drehen_Links [order 3] : [Kran_Drehen_Links  && Kran_Runterlassen]
  Bauteil_Lager_2_Schieben -> Bauteil_Lager_2_Beginnt : [BT_X_Achse <= -2.7]
  Bauteil_Kran_Runterlassen_Und_Drehen_Rechts -> (junction 172) [order 1]
  Bauteil_Lager_3_Beginnt -> Bauteil_Lager_3_Ende : [BT_Z_Achse <= (-19.05 + Lager_3_Status)]
  Bauteil_Kran_Hochheben_Und_Drehen_Rechts -> Bauteil_Kran_Runterlassen_Und_Drehen_Rechts [order 3] : [Kran_Drehen_Rechts  && Kran_Runterlassen]
  Bauteil_Kran_Runterlassen_Und_Drehen_Rechts -> Bauteil_Kran_Hochheben_Und_Drehen_Rechts [order 3] : [Kran_Drehen_Rechts  && Kran_Hochheben]
  Bauteil_Kran_Hochheben_Und_Drehen_Rechts -> (junction 172) [order 1]
  Bauteil_Kran_Hochheben_Und_Drehen_Links -> (junction 172) [order 1]
  Bauteil_Kran_Hochheben_Und_Drehen_Links -> Bauteil_Kran_Runterlassen_Und_Drehen_Links [order 3] : [Kran_Drehen_Links  && Kran_Runterlassen]
  Bauteil_Kran_Runterlassen_Und_Drehen_Links -> Bauteil_Kran_Hochheben_Und_Drehen_Links [order 3] : [Kran_Drehen_Links  && Kran_Hochheben]
  Bauteil_Kran_Runterlassen_Und_Drehen_Links -> (junction 172) [order 1]
  data: Achse function_input double; Schrittgroesse function_input double; MaxWert function_input double; Ausgabe function_output double; Achse function_input double; Schrittgroesse function_input double; MinWert function_input double; Ausgabe function_output double; Lager_Status function_input double; Pos_1 function_input double; Pos_2 function_input double; Ausgabe function_output double; Pos_3 function_input double; BT_Y_Achse output double; BT_Lager output double; Kran_Sauger_BT output double; BT_Bereit output double; BT_X_Achse output double; BT_Z_Achse output double; x local double; Lager_X_Achse input; Lager_Ver_Eingefahren input; Lager_Ver_Ausgefahren input; Kran_Stellung_Lager input; Kran_Stellung_Band input; Kran_Stellung_Stempel input; Kran_Zyl_Oben input; Kran_Zyl_Unten input; Kran_Sauger input; Kran_Hochheben input; Kran_Runterlassen input; Kran_Drehen_Links input; Kran_Drehen_Rechts input; Stempel_Halterung_Ausfahren input; Stempel_Halterung_Einfahren input; Band_Vor input; Band_Zurueck input; Band_Zyl_1_X_Achse input; Band_Zyl_2_X_Achse input; BT_Rotation_1 output double; BT_Rotation_2 output double; BT_Rotation_3 output double; BT_Rotation_4 output double; Lager_Ver_Ausfahren input; Lager_Vereinzler_Schritt_Aus input; Kran_Zyl_Schritt_Hoch input; Kran_Zyl_Schritt_Runter input; Kran_Drehen_Schritt input; Stempel_Halterung_Schritt_Aus input; Stempel_Halterung_Schritt_Ein input; Band_Zyl_1_Schritt input; Band_Zyl_2_Schritt input double; Band_Geschwindigkeit input; Bauteil_Fallgeschwindigkeit input double; Lager_1_Status input; Lager_2_Status input; Lager_3_Status input; Naechste_Position local double; BT_1_Bereit input; BT_2_Bereit input; BT_3_Bereit input; BT_4_Bereit input; BT_5_Bereit input; BT_6_Bereit input; BT_7_Bereit input; BT_8_Bereit input
